simulink library "Px4Library"  (R2015b)
settings: Solver=VariableStepAuto  StartTime=0.0  StopTime=10.0  RelTol=1e-3
undefined symbols (not defined in the file): armed, ctrl_state, INIT_PARAM_VECTOR, mpc_att_sp, mpc_ctrl_state, mpc_manual, mpc_pos_sp_triplet, mpc_vehicle_land_detected, mpc_vehicle_status, v_att_sp, v_control_mode
libraries: simulink x4
(part 1 of 7)
settings Model: Creator=jeremiebannwarth  LastModifiedBy=jban039

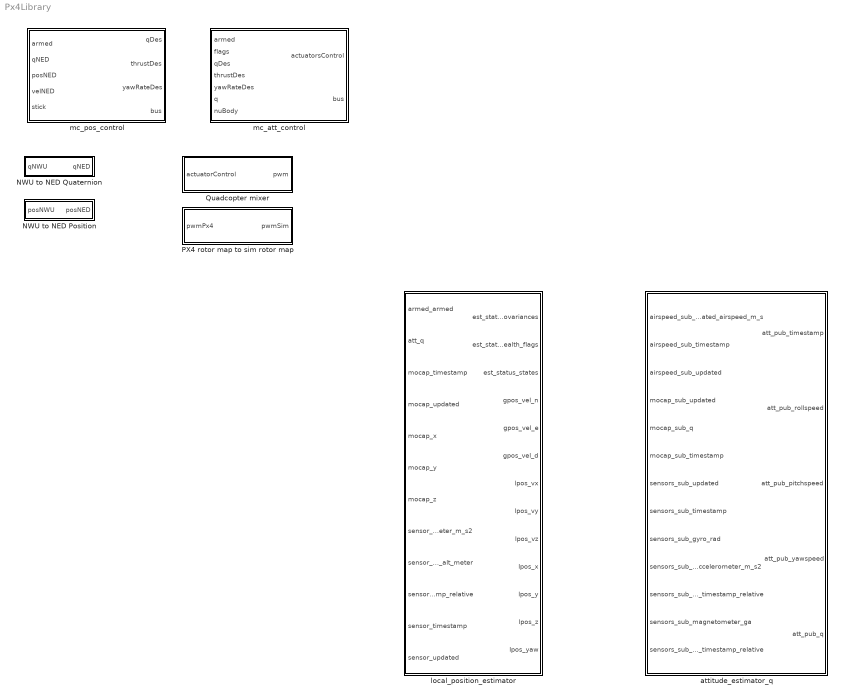
== system Px4Library ==
  NWU to NED Position : Subsystem  mask(Coordinate transform){}
      mask help:
      | Convert a 3x1 vector or 4x1 quaternion from a North West Up to a North East Down coordinate system.
      |
      | The appropriate coordinate transform is automatically selected based on the input size.
  NWU to NED Quaternion : Subsystem  mask(Coordinate transform){}
      mask help:
      | Convert a 3x1 vector or 4x1 quaternion from a North West Up to a North East Down coordinate system.
      |
      | The appropriate coordinate transform is automatically selected based on the input size.
  PX4 rotor map to sim rotor map : Subsystem
      mask Display:
      | disp(sprintf('MOTOR\nMAP'))
      | port_label('output', 1, sprintf('sim\npwm'))
      | port_label('input', 1, sprintf('px4\npwm'))
  Quadcopter mixer : Subsystem  mask{MC_SAMPLING_PERIOD=0.002}
      mask Display:
      | disp('MIXER')
      | port_label('input', 1, sprintf('actuators\ncontrol'))
      | port_label('output', 1, sprintf('px4\npwm'))
  attitude_estimator_q : Subsystem  mask(PX4 LPE (local position estimator): local_position_estimator){Q_SAMPLING_PERIOD=0.002, ATT_W_ACC=0.2, ATT_W_MAG=0.1, ATT_W_EXT_HDG=0.1, ATT_W_GYRO_BIAS=0.1, ATT_MAG_DECL=0, ATT_MAG_DECL_A=1, ATT_EXT_HDG_M=0, ATT_ACC_COMP=1, ATT_BIAS_MAX=0.05, FW_ARSP_MODE=0}
      mask prompts: Q_SAMPLING_PERIOD "Sampling period (s)"; ATT_W_ACC "ATT_W_ACC - Complimentary filter accelerometer weight (-)"; ATT_W_MAG "ATT_W_MAG - Complimentary filter magnetometer weight (-)"; ATT_W_EXT_HDG "ATT_W_EXT_HDG - Complimentary filter external heading weight (-)"; ATT_W_GYRO_BIAS "ATT_W_GYRO_BIAS - Complimentary filter gyroscope bias weight (-)"; ATT_MAG_DECL "ATT_MAG_DECL - Magnetic declination. Not used when GPS available (deg)"; ATT_MAG_DECL_A "ATT_MAG_DECL_A - Automatic GPS based declination compensation (-)"; ATT_EXT_HDG_M "ATT_EXT_HDG_M - External heading usage mode (from Motion capture/Vision) (-), 0 None 1 Vision 2 Motion Capture"; ATT_ACC_COMP "ATT_ACC_COMP - Acceleration compensation based on GPS velocity. (-)"; ATT_BIAS_MAX "ATT_BIAS_MAX - Gyro bias limit (rad/s)"; FW_ARSP_MODE "FW_ARSP_MODE - Method used to publish the airspeed (-), 0 Measured airspeed 1 Vehicle ground speed 2 Airspeed invalid"
      mask TypeOptions ATT_EXT_HDG_M: 0 | 1 | 2
      mask TypeOptions FW_ARSP_MODE: 0 | 1 | 2
  local_position_estimator : Subsystem  mask(PX4 LPE (local position estimator): local_position_estimator){LPE_SAMPLING_PERIOD=0.02, ATT_W_ACC=0.2, Barometer=off, GPS=off, LIDAR=off, Flow=off, Sonar=off, Vision=off, Mocap=off, Land=off}
      mask prompts: LPE_SAMPLING_PERIOD "Sampling period (s)"; ATT_W_ACC "ATT_W_ACC - Complimentary filter accelerometer weight (-)"; Barometer "Use Barometer"; GPS "Use GPS"; LIDAR "Use LIDAR"; Flow "Use Flow"; Sonar "Use Sonar"; Vision "Use Vision"; Mocap "Use Mocap"; Land "Use Land"
      mask Callback Barometer:
      | status = get_param( gcb, 'Barometer' );
      | if strcmp( status, 'on' )
      | 	lpe = bitor( uint8(str2num(get_param( gcb, 'LPE_FUSION' ))), uint8(2^0) );
      | 	set_param( gcb, 'LPE_FUSION', num2str(lpe) );
      | else
      | 	lpe = bitand( uint8(str2num(get_param( gcb, 'LPE_FUSION' ))), bitcmp(uint8(2^0), 'uint8' ));
      | 	set_param( gcb, 'LPE_FUSION', num2str(lpe) );
      | end
      mask Callback GPS:
      | status = get_param( gcb, 'GPS' );
      | if strcmp( status, 'on' )
      | 	lpe = bitor( uint8(str2num(get_param( gcb, 'LPE_FUSION' ))), uint8(2^1) );
      | 	set_param( gcb, 'LPE_FUSION', num2str(lpe) );
      | else
      | 	lpe = bitand( uint8(str2num(get_param( gcb, 'LPE_FUSION' ))), bitcmp(uint8(2^1), 'uint8' ));
      | 	set_param( gcb, 'LPE_FUSION', num2str(lpe) );
      | end
      mask Callback LIDAR:
      | status = get_param( gcb, 'LIDAR' );
      | if strcmp( status, 'on' )
      | 	lpe = bitor( uint8(str2num(get_param( gcb, 'LPE_FUSION' ))), uint8(2^2) );
      | 	set_param( gcb, 'LPE_FUSION', num2str(lpe) );
      | else
      | 	lpe = bitand( uint8(str2num(get_param( gcb, 'LPE_FUSION' ))), bitcmp(uint8(2^2), 'uint8' ));
      | 	set_param( gcb, 'LPE_FUSION', num2str(lpe) );
      | end
      mask Callback Flow:
      | status = get_param( gcb, 'Flow' );
      | if strcmp( status, 'on' )
      | 	lpe = bitor( uint8(str2num(get_param( gcb, 'LPE_FUSION' ))), uint8(2^3) );
      | 	set_param( gcb, 'LPE_FUSION', num2str(lpe) );
      | else
      | 	lpe = bitand( uint8(str2num(get_param( gcb, 'LPE_FUSION' ))), bitcmp(uint8(2^3), 'uint8' ));
      | 	set_param( gcb, 'LPE_FUSION', num2str(lpe) );
      | end
      mask Callback Sonar:
      | status = get_param( gcb, 'Sonar' );
      | if strcmp( status, 'on' )
      | 	lpe = bitor( uint8(str2num(get_param( gcb, 'LPE_FUSION' ))), uint8(2^4) );
      | 	set_param( gcb, 'LPE_FUSION', num2str(lpe) );
      | else
      | 	lpe = bitand( uint8(str2num(get_param( gcb, 'LPE_FUSION' ))), bitcmp(uint8(2^4), 'uint8' ));
      | 	set_param( gcb, 'LPE_FUSION', num2str(lpe) );
      | end
      mask Callback Vision:
      | status = get_param( gcb, 'Vision' );
      | if strcmp( status, 'on' )
      | 	lpe = bitor( uint8(str2num(get_param( gcb, 'LPE_FUSION' ))), uint8(2^5) );
      | 	set_param( gcb, 'LPE_FUSION', num2str(lpe) );
      | else
      | 	lpe = bitand( uint8(str2num(get_param( gcb, 'LPE_FUSION' ))), bitcmp(uint8(2^5), 'uint8' ));
      | 	set_param( gcb, 'LPE_FUSION', num2str(lpe) );
      | end
      mask Callback Mocap:
      | status = get_param( gcb, 'Mocap' );
      | if strcmp( status, 'on' )
      | 	lpe = bitor( uint8(str2num(get_param( gcb, 'LPE_FUSION' ))), uint8(2^6) );
      | 	set_param( gcb, 'LPE_FUSION', num2str(lpe) );
      | else
      | 	lpe = bitand( uint8(str2num(get_param( gcb, 'LPE_FUSION' ))), bitcmp(uint8(2^6), 'uint8' ));
      | 	set_param( gcb, 'LPE_FUSION', num2str(lpe) );
      | end
      mask Callback Land:
      | status = get_param( gcb, 'Land' );
      | if strcmp( status, 'on' )
      | 	lpe = bitor( uint8(str2num(get_param( gcb, 'LPE_FUSION' ))), uint8(2^7) );
      | 	set_param( gcb, 'LPE_FUSION', num2str(lpe) );
      | else
      | 	lpe = bitand( uint8(str2num(get_param( gcb, 'LPE_FUSION' ))), bitcmp(uint8(2^7), 'uint8' ));
      | 	set_param( gcb, 'LPE_FUSION', num2str(lpe) );
      | end
  mc_att_control : Subsystem  mask(PX4 Attitude Controller: mc_att_control){MC_SAMPLING_PERIOD=0.002, MC_ROLL_TC=0.2, MC_PITCH_TC=0.2, MC_ROLL_P=6.5, MC_ROLLRATE_P=0.15, MC_ROLLRATE_I=0.05, MC_ROLLRATE_D=0.003, MC_ROLLRATE_FF=0.0, MC_PITCH_P=6.5, MC_PITCHRATE_P=0.15, MC_PITCHRATE_I=0.05, MC_PITCHRATE_D=0.003, MC_PITCHRATE_FF=0.0, MC_YAW_P=2.8, MC_YAWRATE_P=0.2, MC_YAWRATE_I=0.1, MC_YAWRATE_D=0.0, MC_YAWRATE_FF=0.0, MC_YAW_FF=0.5, MC_ROLLRATE_MAX=220.0, MC_PITCHRATE_MAX=220.0, MC_YAWRATE_MAX=200.0, MC_YAWRAUTO_MAX=45.0, MC_ACRO_R_MAX=360.0, MC_ACRO_P_MAX=360.0, MC_ACRO_Y_MAX=360.0, MC_RATT_TH=0.8, MC_TPA_BREAK=1.0, MC_TPA_SLOPE=1.0, VT_OPT_RECOV_EN=0.0, VT_WV_YAWR_SCL=0.15, MC_RR_INT_LIM=0.30, MC_PR_INT_LIM=0.30, MC_TPA_BREAK_P=1.0, MC_TPA_BREAK_I=1.0, MC_TPA_BREAK_D=1.0, MC_TPA_RATE_P=0.0, MC_TPA_RATE_I=0.0, MC_TPA_RATE_D=0.0, VT_TYPE=2.0, MC_BAT_SCALE_EN=0.0, MC_YR_INT_LIM=0.30}
      mask prompts: VT_TYPE "VT_TYPE (0 = Tailsitter, 1 = Tiltrotor, 2 = Standard)"
      mask help: Stabilization controller from the PX4 flight stack.
  mc_pos_control : Subsystem  mask{THROTTLE_HOVER=0.61703684833922, MPC_SAMPLING_PERIOD=0.02, MPC_THR_MIN=0.12, MPC_THR_HOVER=0.5, MPC_ALTCTL_DZ=0.1, MPC_ALTCTL_DY=0.0, MPC_THR_MAX=0.9, MPC_MANTHR_MIN=0.08, MPC_MANTHR_MAX=0.9, MPC_Z_P=1.0, MPC_Z_VEL_P=0.2, MPC_Z_VEL_I=0.02, MPC_Z_VEL_D=0.0, MPC_Z_VEL_MAX_UP=3.0, MPC_Z_VEL_MAX=1.0, MPC_Z_VEL_MAX_DN=1.0, MPC_Z_FF=0.5, MPC_XY_P=0.95, MPC_XY_VEL_P=0.09, MPC_XY_VEL_I=0.02, MPC_XY_VEL_D=0.01, MPC_XY_CRUISE=5.0, MPC_XY_VEL_MAX=8.0, MPC_XY_FF=0.5, MPC_TILTMAX_AIR=45.0, MPC_TILTMAX_LND=12.0, MPC_LAND_SPEED=0.5, MPC_TKO_SPEED=1.5, MPC_MAN_R_MAX=35.0, MPC_MAN_P_MAX=35.0, MPC_MAN_Y_MAX=200.0, MPC_HOLD_XY_DZ=0.1, MPC_HOLD_MAX_XY=0.8, MPC_HOLD_MAX_Z=0.6, MPC_VELD_LP=5.0, MPC_ACC_HOR_MAX=5.0, MPC_ALT_MODE=0, MC_YAWRATE_MAX=200.0, MC_YAW_P=2.8, VT_OPT_RECOV_EN=0}
      mask init:
      | throttle_hover = THROTTLE_HOVER; % evalin('base', THROTTLE_HOVER);
      | MPC_INIT_SELF = struct( 'mpc_param_find', struct( ...
      | 'MC_YAWRATE_MAX', str2num(MC_YAWRATE_MAX), ...
      | 'MC_YAW_P', str2num(MC_YAW_P), ...
      | 'MPC_ACC_HOR_MAX', str2num(MPC_ACC_HOR_MAX), ...
      | 'MPC_ALTCTL_DY', str2num(MPC_ALTCTL_DY), ...
      | 'MPC_ALTCTL_DZ', str2num(MPC_ALTCTL_DZ), ...
      | 'MPC_ALT_MODE', str2num(MPC_ALT_MODE), ...
      | 'MPC_HOLD_MAX_XY', str2num(MPC_HOLD_MAX_XY), ...
      | 'MPC_HOLD_MAX_Z', str2num(MPC_HOLD_MAX_Z), ...
      | 'MPC_HOLD_XY_DZ', str2num(MPC_HOLD_XY_DZ), ...
      | 'MPC_LAND_SPEED', str2num(MPC_LAND_SPEED), ...
      | 'MPC_MAN_P_MAX', str2num(MPC_MAN_P_MAX), ...
      | 'MPC_MAN_R_MAX', str2num(MPC_MAN_R_MAX), ...
      | 'MPC_MAN_Y_MAX', str2num(MPC_MAN_Y_MAX), ...
      | 'MPC_THR_HOVER', str2num(MPC_THR_HOVER), ...
      | 'MPC_THR_MAX', str2num(MPC_THR_MAX), ...
      | 'MPC_THR_MIN', str2num(MPC_THR_MIN), ...
      | 'MPC_TILTMAX_AIR', str2num(MPC_TILTMAX_AIR), ...
      | 'MPC_TILTMAX_LND', str2num(MPC_TILTMAX_LND), ...
      | 'MPC_TKO_SPEED', str2num(MPC_TKO_SPEED), ...
      | 'MPC_XY_CRUISE', str2num(MPC_XY_CRUISE), ...
      | 'MPC_XY_FF', str2num(MPC_XY_FF), ...
      | 'MPC_XY_P', str2num(MPC_XY_P), ...
      | 'MPC_XY_VEL_D', str2num(MPC_XY_VEL_D), ...
      | 'MPC_XY_VEL_I', str2num(MPC_XY_VEL_I), ...
      | 'MPC_XY_VEL_MAX', str2num(MPC_XY_VEL_MAX), ...
      | 'MPC_XY_VEL_P', str2num(MPC_XY_VEL_P), ...
      | 'MPC_Z_FF', str2num(MPC_Z_FF), ...
      | 'MPC_Z_P', str2num(MPC_Z_P), ...
      | 'MPC_Z_VEL_D', str2num(MPC_Z_VEL_D), ...
      | 'MPC_Z_VEL_I', str2num(MPC_Z_VEL_I), ...
      | 'MPC_Z_VEL_MAX', str2num(MPC_Z_VEL_MAX), ...
      | 'MPC_Z_VEL_MAX_DN', str2num(MPC_Z_VEL_MAX_DN), ...
      | 'MPC_Z_VEL_MAX_UP', str2num(MPC_Z_VEL_MAX_UP), ...
      | 'MPC_Z_VEL_P', str2num(MPC_Z_VEL_P), ...
      | 'VT_OPT_RECOV_EN', str2num(VT_OPT_RECOV_EN), ...
      | 'MPC_VELD_LP', str2num(MPC_VELD_LP) ...
      | ), ...
      | 'mpc_thrust_int', [0; 0; -throttle_hover], ...
      | 'mpc_att_sp', struct('thrust', throttle_hover, ...
      | 'q_d', [1; 0; 0; 0;]) ...
      | );

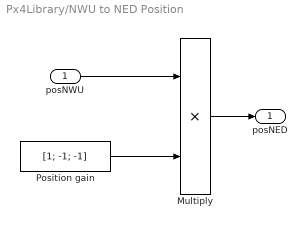
== system Px4Library/NWU to NED Position ==
  posNWU : Inport
  Multiply : Product  Inputs=**
  Position gain : Constant  Value=[1; -1; -1]
  posNED : Outport
  wires:
  Position gain/1 -> Multiply/2
  Multiply/1 -> posNED/1
  posNWU/1 -> Multiply/1

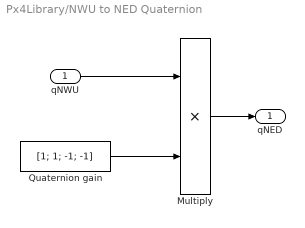
== system Px4Library/NWU to NED Quaternion ==
  qNWU : Inport
  Multiply : Product  Inputs=**
  Quaternion gain : Constant  Value=[1; 1; -1; -1]
  qNED : Outport
  wires:
  qNWU/1 -> Multiply/1
  Multiply/1 -> qNED/1
  Quaternion gain/1 -> Multiply/2

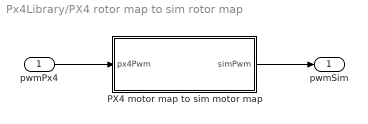
== system Px4Library/PX4 rotor map to sim rotor map ==
  pwmPx4 : Inport
  PX4 motor map to sim motor map : MATLAB Function  TreatAsAtomicUnit=on
  pwmSim : Outport
  wires:
  PX4 motor map to sim motor map/1(simPwm) -> pwmSim/1
  pwmPx4/1 -> PX4 motor map to sim motor map/1(px4Pwm)

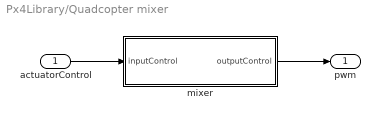
== system Px4Library/Quadcopter mixer ==
  actuatorControl : Inport
  mixer : MATLAB Function  TreatAsAtomicUnit=on  SystemSampleTime=MC_SAMPLING_PERIOD
  pwm : Outport
  wires:
  actuatorControl/1 -> mixer/1(inputControl)
  mixer/1(outputControl) -> pwm/1

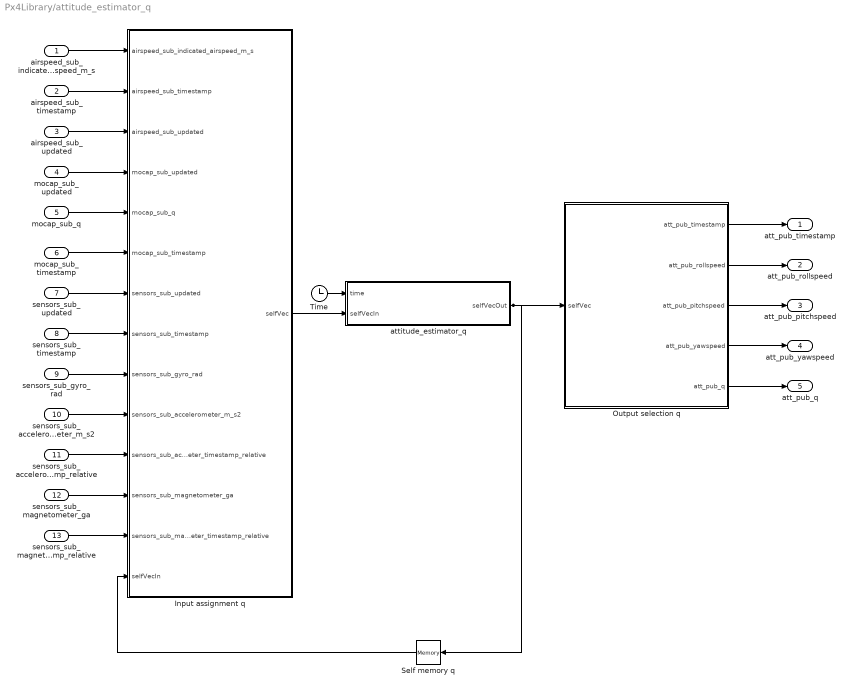
== system Px4Library/attitude_estimator_q ==
  airspeed_sub_indicated_airspeed_m_s : Inport
  airspeed_sub_timestamp : Inport  Port=2
  airspeed_sub_updated : Inport  Port=3
  mocap_sub_updated : Inport  Port=4
  mocap_sub_q : Inport  Port=5
  mocap_sub_timestamp : Inport  Port=6
  sensors_sub_updated : Inport  Port=7
  sensors_sub_timestamp : Inport  Port=8
  sensors_sub_gyro_rad : Inport  Port=9
  sensors_sub_accelerometer_m_s2 : Inport  Port=10
  sensors_sub_accelerometer_timestamp_relative : Inport  Port=11
  sensors_sub_magnetometer_ga : Inport  Port=12
  sensors_sub_magnetometer_timestamp_relative : Inport  Port=13
  Input assignment q : MATLAB Function  TreatAsAtomicUnit=on
  Output selection q : MATLAB Function  TreatAsAtomicUnit=on
  Self memory q : Memory  X0=[ATT_ACC_COMP, 0, 0, 0, 0, 0, 0, FW_ARSP_MODE, 0, 0, 0, 0, 0, 0, 0, 0, 0, 0, 0, ATT_BIAS_MAX, 0, 0, 0, 0, 0, 0, 0, 0, 0, 0, 0, 0, 0, 0, 0, 0, 0, 0, 0.02, 0, ATT_EXT_HDG_M, 0, 0, 0, 0, 0, 0, 0, 0, 0, 0, 0, 0, 0, 0, 0, 0, 0, 0, 0, 0, 0, 0, 0, 0, 0, 0, 0, 0, 0, 0, 0, 0, 0, 0, 0, 0, 0, 0, 0, 0, 0, 0, 0, 0, 0, 0, 0, 0, 0, 0, 0, 0, 0, 0, 0, 0, 0, 0, 0, 0, 0, 0, 0, 0, 0, 0, 0, 0, 0, 0, 0, 0, 0, 0, 0, 0, 0, 0, 0, 0, 0, ATT_MAG_DECL, ATT_MAG_DECL_A, 0, 0, 0, 0, 0, 0, 0, 0, 0, 0, 0, 0, 0, 0, 0, 0, 0, 0, 0, 0, 0, 0, 0, 0, 0, 0, 0, 0, 0, 0, 0, 0, 0, 0, 0, 0, 0, 0, 0, 0, 0, 0, 0, 0, 0, 0, 0, 0, 0, 0, 0, 0, 0, 0, 0, 0, 0, 0, 0, 0, ATT_W_ACC, ATT_W_EXT_HDG, ATT_W_GYRO_BIAS, ATT_W_MAG, 0, 0]
  Time : Clock
  attitude_estimator_q : MATLAB Function  TreatAsAtomicUnit=on  SystemSampleTime=Q_SAMPLING_PERIOD
  att_pub_timestamp : Outport
  att_pub_rollspeed : Outport  Port=2
  att_pub_pitchspeed : Outport  Port=3
  att_pub_yawspeed : Outport  Port=4
  att_pub_q : Outport  Port=5
  wires:
  Input assignment q/1(selfVec) -> attitude_estimator_q/2(selfVecIn)
  attitude_estimator_q/1(selfVecOut) -> Output selection q/1(selfVec), Self memory q/1
  Self memory q/1 -> Input assignment q/14(selfVecIn)
  Time/1 -> attitude_estimator_q/1(time)
  airspeed_sub_indicated_airspeed_m_s/1 -> Input assignment q/1(airspeed_sub_indicated_airspeed_m_s)
  airspeed_sub_timestamp/1 -> Input assignment q/2(airspeed_sub_timestamp)
  airspeed_sub_updated/1 -> Input assignment q/3(airspeed_sub_updated)
  mocap_sub_updated/1 -> Input assignment q/4(mocap_sub_updated)
  mocap_sub_q/1 -> Input assignment q/5(mocap_sub_q)
  mocap_sub_timestamp/1 -> Input assignment q/6(mocap_sub_timestamp)
  sensors_sub_updated/1 -> Input assignment q/7(sensors_sub_updated)
  sensors_sub_timestamp/1 -> Input assignment q/8(sensors_sub_timestamp)
  sensors_sub_gyro_rad/1 -> Input assignment q/9(sensors_sub_gyro_rad)
  sensors_sub_accelerometer_m_s2/1 -> Input assignment q/10(sensors_sub_accelerometer_m_s2)
  sensors_sub_accelerometer_timestamp_relative/1 -> Input assignment q/11(sensors_sub_accelerometer_timestamp_relative)
  sensors_sub_magnetometer_ga/1 -> Input assignment q/12(sensors_sub_magnetometer_ga)
  sensors_sub_magnetometer_timestamp_relative/1 -> Input assignment q/13(sensors_sub_magnetometer_timestamp_relative)
  Output selection q/1(att_pub_timestamp) -> att_pub_timestamp/1
  Output selection q/2(att_pub_rollspeed) -> att_pub_rollspeed/1
  Output selection q/3(att_pub_pitchspeed) -> att_pub_pitchspeed/1
  Output selection q/4(att_pub_yawspeed) -> att_pub_yawspeed/1
  Output selection q/5(att_pub_q) -> att_pub_q/1

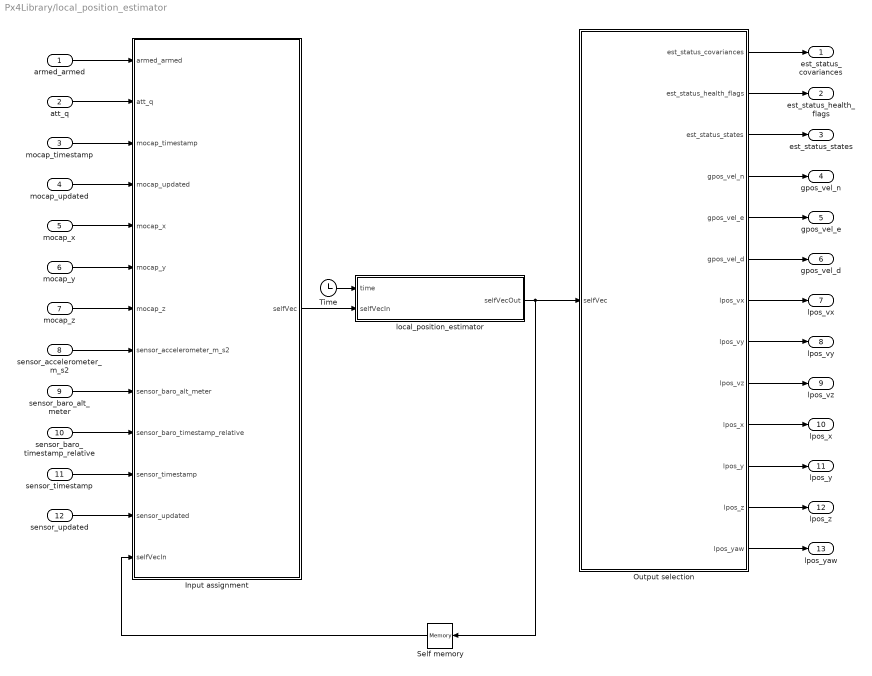
== system Px4Library/local_position_estimator ==
  armed_armed : Inport
  att_q : Inport  Port=2
  mocap_timestamp : Inport  Port=3
  mocap_updated : Inport  Port=4
  mocap_x : Inport  Port=5
  mocap_y : Inport  Port=6
  mocap_z : Inport  Port=7
  sensor_accelerometer_m_s2 : Inport  Port=8
  sensor_baro_alt_meter : Inport  Port=9
  sensor_baro_timestamp_relative : Inport  Port=10
  sensor_timestamp : Inport  Port=11
  sensor_updated : Inport  Port=12
  Input assignment : MATLAB Function  TreatAsAtomicUnit=on
  Output selection : MATLAB Function  TreatAsAtomicUnit=on
  Self memory : Memory  X0=[0, 0, 0, 0, 0, 0, 0, 0, 0, 0, 0, 0, 0, 0, 0, 0, 0, 0, 0, 0, 0, 0, 0, 0, 0, 0, 0, 0, 0, 0, 0, 0, 0, 0, 0, 0, 0, 0, 0, 0, 0, 0, 0, 0, 0, 0, 0, 0, 0, 0, 0, 0, 0, 0, 0, 0, 0, 0, 0, 0, 0, 0, 0, 0, 0, 0, 0, 0, 0, 0, 0, 0, 0, 0, 0, 0, 0, 0, 0, 0, 0, 0, 0, 0, 0, 0, 0, 0, 0, 0, 0, 0, 0, 0, 0, 0, 0, 0, 0, 0, 0, 0, 0, 0, 0, 0, 0, 0, 0, 0, 0, 0, 0, 0, 0, 0, 0, 0, 0, 0, 0, 0, 0, 0, 0, 0, 0, 0, 0, 0, 0, 8.82050518214, 12.094592431, 13.9876612368, 16.0875642296, 17.8797700658, 19.6465647819, 1e-1, 2.0, 2.0, 2.0, 2^2, 2^0, 2^1, 2^7, 2^1, 2^6, 2^0, 2^4, 2^5, 2^2, 2^3, 0, 10.0, 8, 0, 0, 0, 0, 0, 0, 0, 0, 0, 0, 8, 0, 0, 0, 0, 0, 0, 0, 0, 0, 0, 8, 0, 0, 0, 0, 0, 0, 0, 0, 0, 0, 2*LPE_VXY_PUB*LPE_VXY_PUB, 0, 0, 0, 0, 0, 0, 0, 0, 0, 0, 2*LPE_VXY_PUB*LPE_VXY_PUB, 0, 0, 0, 0, 0, 0, 0, 0, 0, 0, 2*LPE_VXY_PUB*LPE_VXY_PUB, 0, 0, 0, 0, 0, 0, 0, 0, 0, 0, 1e-6, 0, 0, 0, 0, 0, 0, 0, 0, 0, 0, 1e-6, 0, 0, 0, 0, 0, 0, 0, 0, 0, 0, 1e-6, 0, 0, 0, 0, 0, 0, 0, 0, 0, 0, 8, 1.0e6, 0, 0, 0, 0, 0, 0, 0, 0, 0, 0, 0, 0, 0, 0, 0, 0, 0, 0, 0, 0, 0, 0, 0, 0, 0, 0, 0, 0, 0, 0, 0, 0, 0, 0, 0, 0, 0, 0, 0, 0, 0, 0, 0, 0, 0, 0, 0, 0, 0, 0, 0, 0, 0, 0, 0, 0, 0, 0, 0, 0, 0, 0, 0, 0, 0, 0, 0, 0, 0, 0, 0, 0, 0, 0, 0, 0, 0, 0, 0, 0, 0, 0, 0, 0, 0, 0, 0, 0, 0, 0, 0, 0, 0, 0, 0, 0, 0, 0, 0, 0, 0, 0, 0, 0, 0, 0, 0, 0, 0, 0, 0, 0, 0, 0, 0, 0, 0, 0, 2^0, 2^3, 2^1, 2^7, 2^2, 2^6, 2^4, 2^5, 0, LPE_ACC_XY, 0, LPE_ACC_Z, LPE_SAMPLING_PERIOD, LPE_X_LP, 0, 0, 0, 0, 0, 0, LPE_BAR_Z, LPE_SAMPLING_PERIOD, 0, 0, 0, 0, LPE_FAKE_ORIGIN, 0, LPE_FGYRO_HP, LPE_FGYRO_HP, LPE_FLW_QMIN, LPE_FLW_R, LPE_FLW_RR, LPE_FLW_SCALE, LPE_FLW_OFF_Z, LPE_FUSION, 0, LPE_GPS_DELAY, LPE_EPH_MAX, LPE_EPV_MAX, LPE_GPS_VXY, LPE_GPS_VZ, LPE_GPS_XY, LPE_GPS_Z, LPE_LAT, LPE_LON, 0, 0, LPE_LAND_VXY, LPE_LAND_Z, 0, LPE_LDR_OFF_Z, LPE_LDR_Z, 0, 0, 0, 0, 0, 0, 0, LPE_VIC_P, LPE_PN_B, LPE_PN_P, LPE_PN_T, LPE_PN_V, 8, 0, 0, 0, 0, 0, 0, 0, 0, 0, 0, 0, 0, 0, 0, 0, 0, 0, 0, 0, 0, 0, 0, 0, 0, 0, 0, 0, 0, 0, 0, 0, 0, 0, 0, 0, 0, 0, 0, 0, 0, 0, 0, 0, 0, 0, 0, 0, 0, 0, 0, 0, 0, 0, 0, 0, 0, 0, 0, 0, 0, 0, 0, 0, 0, 0, 0, 0, 0, 0, 0, 0, 0, 0, 0, 255, 0, LPE_SNR_OFF_Z, LPE_SNR_Z, 0, 0, 0, 0, 0, 0, 0, 0, 0, 0, 0, 0, 0, 0, 0, 0, 0, 0, 0, 0, 0, 0, 0, 0, 0, 0, 0, 0, 0, 0, 0, 0, 0, 0, 0, 0, 0, 0, 0, 1, 1, LPE_T_MAX_GRADE, 0, 0, 0, 0, 0, 0, 0, 0, 0, 0, 0, LPE_VIS_DELAY, LPE_VIS_XY, LPE_VIS_Z, LPE_VXY_PUB, 0, 0, 0, 0, 0, 0, 0, 0, 0, 0, 0, 0, 0, 0, 0, 0, 0, 0, 0, 0, 0, 0, 0, 0, 0, 0, 0, 0, 0, 0, 0, 0, 0, 0, 0, 0, 0, 0, 0, 0, 0, 0, 0, 0, 0, 0, 0, 0, 0, 0, 0, 0, 0, 0, 0, 0, 0, 0, 0, 0, 0, 0, 0, 0, 0, 0, 0, 0, 0, 0, 0, 0, 0, 0, 0, 0, 0, 0, 0, 0, 0, 0, 0, 0, 0, 0, 0, 0, 0, 0, 0, 0, 0, 0, 0, 0, 0, 0, 0, 0, 0, 0, 0, 0, 0, 0, 0, 0, 0, 0, 1, 1, LPE_SAMPLING_PERIOD, LPE_X_LP, 0, 0, 0, 0, 0, 0, 0, 0, 0, 0, LPE_Z_PUB]
  Time : Clock
  local_position_estimator : MATLAB Function  TreatAsAtomicUnit=on  SystemSampleTime=LPE_SAMPLING_PERIOD
  est_status_covariances : Outport
  est_status_health_flags : Outport  Port=2
  est_status_states : Outport  Port=3
  gpos_vel_n : Outport  Port=4
  gpos_vel_e : Outport  Port=5
  gpos_vel_d : Outport  Port=6
  lpos_vx : Outport  Port=7
  lpos_vy : Outport  Port=8
  lpos_vz : Outport  Port=9
  lpos_x : Outport  Port=10
  lpos_y : Outport  Port=11
  lpos_z : Outport  Port=12
  lpos_yaw : Outport  Port=13
  wires:
  Input assignment/1(selfVec) -> local_position_estimator/2(selfVecIn)
  local_position_estimator/1(selfVecOut) -> Output selection/1(selfVec), Self memory/1
  Self memory/1 -> Input assignment/13(selfVecIn)
  Time/1 -> local_position_estimator/1(time)
  armed_armed/1 -> Input assignment/1(armed_armed)
  att_q/1 -> Input assignment/2(att_q)
  mocap_timestamp/1 -> Input assignment/3(mocap_timestamp)
  mocap_updated/1 -> Input assignment/4(mocap_updated)
  mocap_x/1 -> Input assignment/5(mocap_x)
  mocap_y/1 -> Input assignment/6(mocap_y)
  mocap_z/1 -> Input assignment/7(mocap_z)
  sensor_accelerometer_m_s2/1 -> Input assignment/8(sensor_accelerometer_m_s2)
  sensor_baro_alt_meter/1 -> Input assignment/9(sensor_baro_alt_meter)
  sensor_baro_timestamp_relative/1 -> Input assignment/10(sensor_baro_timestamp_relative)
  sensor_timestamp/1 -> Input assignment/11(sensor_timestamp)
  sensor_updated/1 -> Input assignment/12(sensor_updated)
  Output selection/1(est_status_covariances) -> est_status_covariances/1
  Output selection/2(est_status_health_flags) -> est_status_health_flags/1
  Output selection/3(est_status_states) -> est_status_states/1
  Output selection/4(gpos_vel_n) -> gpos_vel_n/1
  Output selection/5(gpos_vel_e) -> gpos_vel_e/1
  Output selection/6(gpos_vel_d) -> gpos_vel_d/1
  Output selection/7(lpos_vx) -> lpos_vx/1
  Output selection/8(lpos_vy) -> lpos_vy/1
  Output selection/9(lpos_vz) -> lpos_vz/1
  Output selection/10(lpos_x) -> lpos_x/1
  Output selection/11(lpos_y) -> lpos_y/1
  Output selection/12(lpos_z) -> lpos_z/1
  Output selection/13(lpos_yaw) -> lpos_yaw/1

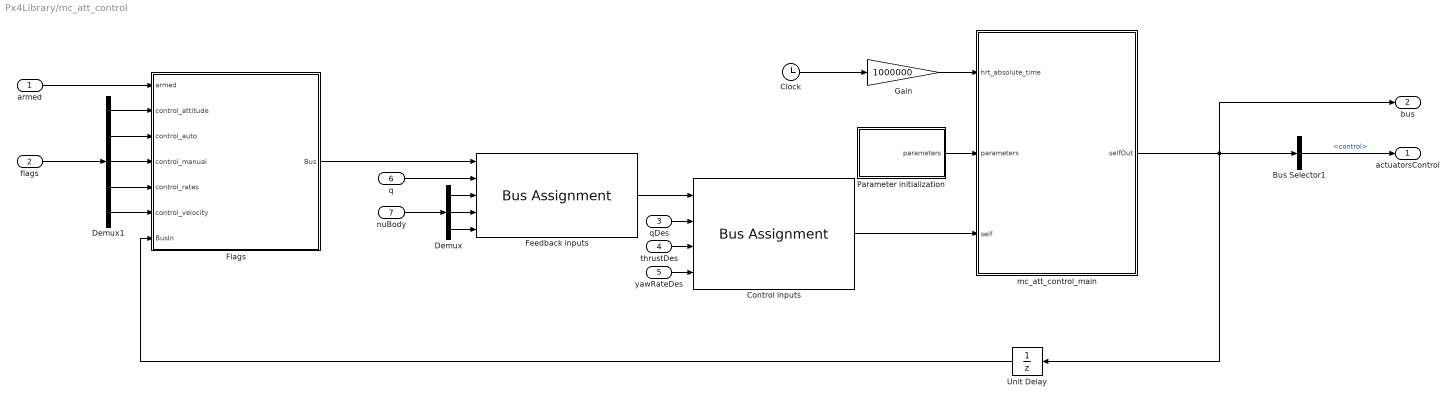
== system Px4Library/mc_att_control ==
  armed : Inport  PortDimensions=1  SampleTime=MC_SAMPLING_PERIOD
  flags : Inport  Port=2  PortDimensions=5  SampleTime=MC_SAMPLING_PERIOD
  qDes : Inport  Port=3  PortDimensions=4  SampleTime=MC_SAMPLING_PERIOD
  thrustDes : Inport  Port=4  PortDimensions=1  SampleTime=MC_SAMPLING_PERIOD
  yawRateDes : Inport  Port=5  PortDimensions=1  SampleTime=MC_SAMPLING_PERIOD
  q : Inport  Port=6  PortDimensions=4  SampleTime=MC_SAMPLING_PERIOD
  nuBody : Inport  Port=7  PortDimensions=3  SampleTime=MC_SAMPLING_PERIOD
  Bus Selector1 : BusSelector  OutputSignals=actuators.control
  Clock : Clock
  Control inputs : BusAssignment  AssignedSignals=v_att_sp.q_d,v_att_sp.thrust,v_att_sp.yaw_sp_move_rate
  Demux : Demux  Outputs=3
  Demux1 : Demux  Outputs=5
  Feedback inputs : BusAssignment  AssignedSignals=ctrl_state.q,ctrl_state.roll_rate,ctrl_state.pitch_rate,ctrl_state.yaw_rate
  Flags : Subsystem
  Gain : Gain  Gain=1000000
  Parameter initialization : Subsystem
  Unit Delay : UnitDelay  SampleTime=MC_SAMPLING_PERIOD
  mc_att_control_main : MATLAB Function  TreatAsAtomicUnit=on  SystemSampleTime=MC_SAMPLING_PERIOD
  actuatorsControl : Outport  SampleTime=MC_SAMPLING_PERIOD
  bus : Outport  Port=2  SampleTime=MC_SAMPLING_PERIOD
  wires:
  mc_att_control_main/1(selfOut) -> bus/1, Unit Delay/1, Bus Selector1/1
  Parameter initialization/1(parameters) -> mc_att_control_main/2(parameters)
  Bus Selector1/1 -> actuatorsControl/1  "<control>"
  Unit Delay/1 -> Flags/7(BusIn)
  Control inputs/1 -> mc_att_control_main/3(self)
  Flags/1(Bus) -> Feedback inputs/1
  Demux/1 -> Feedback inputs/3
  Demux/2 -> Feedback inputs/4
  Demux/3 -> Feedback inputs/5
  Clock/1 -> Gain/1
  Gain/1 -> mc_att_control_main/1(hrt_absolute_time)
  Feedback inputs/1 -> Control inputs/1
  qDes/1 -> Control inputs/2
  thrustDes/1 -> Control inputs/3
  yawRateDes/1 -> Control inputs/4
  Demux1/5 -> Flags/6(control_velocity)
  Demux1/4 -> Flags/5(control_rates)
  Demux1/3 -> Flags/4(control_manual)
  Demux1/2 -> Flags/3(control_auto)
  Demux1/1 -> Flags/2(control_attitude)
  armed/1 -> Flags/1(armed)
  q/1 -> Feedback inputs/2
  nuBody/1 -> Demux/1
  flags/1 -> Demux1/1

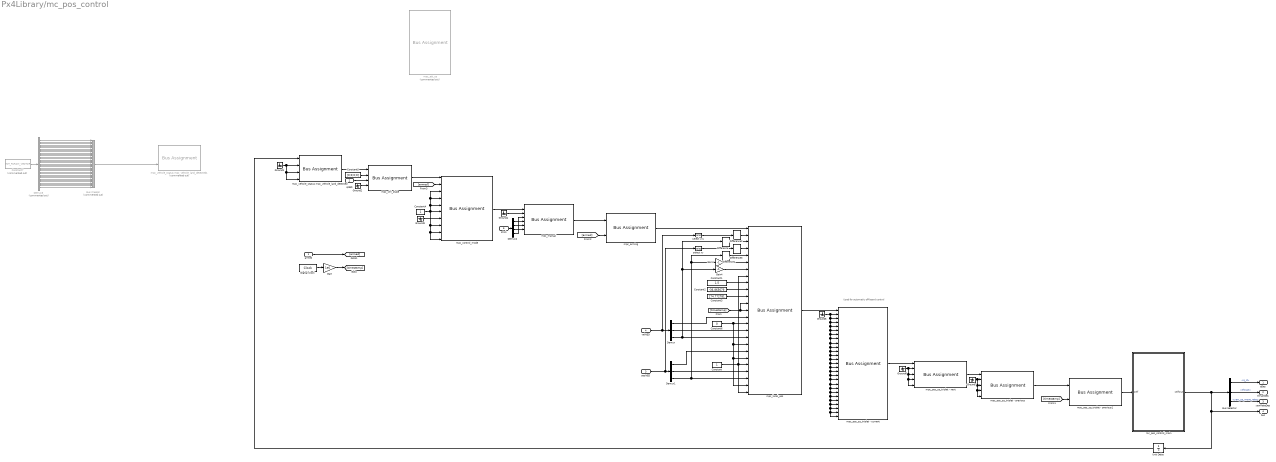
== system Px4Library/mc_pos_control ==
  note: Used for automatic off-board control
  armed : Inport  PortDimensions=1  SampleTime=MPC_SAMPLING_PERIOD
  qNED : Inport  Port=2  PortDimensions=4  SampleTime=MPC_SAMPLING_PERIOD
  posNED : Inport  Port=3  PortDimensions=3  SampleTime=MPC_SAMPLING_PERIOD
  velNED : Inport  Port=4  PortDimensions=3  SampleTime=MPC_SAMPLING_PERIOD
  stick : Inport  Port=5  PortDimensions=4  SampleTime=MPC_SAMPLING_PERIOD
  Bus Creator : BusCreator  Commented=on  Inputs=35  OutDataTypeStr=Bus: mpc_param_find
  Bus Selector : BusSelector  OutputSignals=mpc_att_sp.q_d,mpc_att_sp.thrust,mpc_att_sp.yaw_sp_move_rate
  Constant : Constant  SampleTime=MPC_SAMPLING_PERIOD
  Constant1 : Constant  Value=1.5  SampleTime=MPC_SAMPLING_PERIOD
  Constant2 : Constant  Value=-36.865679  SampleTime=MPC_SAMPLING_PERIOD
  Constant3 : Constant  Value=174.772781  SampleTime=MPC_SAMPLING_PERIOD
  Constant4 : Constant
  Constant5 : Constant  Value=[0;0;0;0]
  Constant6 : Constant  Value=0  SampleTime=MPC_SAMPLING_PERIOD
  Constant7 : Constant  Commented=on  Value=INIT_PARAM_VECTOR
  Demux : Demux  Outputs=3
  Demux1 : Demux  Outputs=3
  Demux2 : Demux
  Demux3 : Demux  Commented=on  Outputs=35
  Difference{,1..3} (4 alike) : simulink/Discrete/Difference  ICPrevInput=0.0  InputProcessing=Inherited  OutMin=[]  OutMax=[]  OutDataType=fixdt(1, 16)  OutScaling=2^-10  DoSatur=off
  Digital Clock : DigitalClock  SampleTime=MPC_SAMPLING_PERIOD
  Gain : Gain  Gain=1e6
  Gain1 : Gain  Gain=-1
  Gain4 : Gain  Gain=-1
  Ground{1..7} (7 alike) : Ground
  Unit Delay : UnitDelay  InitialCondition=MPC_INIT_SELF  SampleTime=MPC_SAMPLING_PERIOD
  mc_pos_control_main : MATLAB Function  TreatAsAtomicUnit=on  SystemSampleTime=MPC_SAMPLING_PERIOD
  mpc_arming : BusAssignment  AssignedSignals=mpc_arming.armed
  mpc_att_sp : BusAssignment  Commented=on  AssignedSignals=mpc_att_sp.disable_mc_yaw_control,mpc_att_sp.landing_gear,mpc_att_sp.pitch_body,mpc_att_sp.q_d,mpc_att_sp.q_d_valid,mpc_att_sp.roll_body,mpc_att_sp.thrust,mpc_att_sp.timestamp,mpc_att_sp.yaw_body,mpc_att_sp.yaw_sp_move_rate
  mpc_control_mode : BusAssignment  AssignedSignals=mpc_control_mode.flag_armed,mpc_control_mode.flag_control_acceleration_enabled,mpc_control_mode.flag_control_altitude_enabled,mpc_control_mode.flag_control_climb_rate_enabled,mpc_control_mode.flag_control_manual_enabled,mpc_control_mode.flag_control_offboard_enabled,mpc_control_mode.flag_control_position_enabled,mpc_control_mode.flag_control_velocity_enabled,mpc_control_mode.flag_control_attitude_enabled
  mpc_ctrl_state : BusAssignment  AssignedSignals=mpc_ctrl_state.delta_q_reset,mpc_ctrl_state.q,mpc_ctrl_state.quat_reset_counter
  mpc_local_pos : BusAssignment  AssignedSignals=mpc_local_pos.delta_vxy,mpc_local_pos.delta_vz,mpc_local_pos.delta_xy,mpc_local_pos.delta_z,mpc_local_pos.dist_bottom,mpc_local_pos.dist_bottom_rate,mpc_local_pos.dist_bottom_valid,mpc_local_pos.ref_alt,mpc_local_pos.ref_lat,mpc_local_pos.ref_lon,mpc_local_pos.ref_timestamp,mpc_local_pos.timestamp,mpc_local_pos.vx,mpc_local_pos.vxy_reset_counter,mpc_local_pos.vy,mpc_local_pos.vz,mpc_local_pos.vz_reset_counter,mpc_local_pos.x,mpc_local_pos.xy_reset_counter,mpc_local_pos.xy_valid,mpc_local_pos.y,mpc_local_pos.z,mpc_local_pos.z_reset_counter,mpc_local_pos.z_valid
  mpc_manual : BusAssignment  AssignedSignals=mpc_manual.gear_switch,mpc_manual.r,mpc_manual.x,mpc_manual.y,mpc_manual.z
  mpc_pos_sp_triplet - current : BusAssignment  AssignedSignals=mpc_pos_sp_triplet.mpc_current.a_x,mpc_pos_sp_triplet.mpc_current.a_y,mpc_pos_sp_triplet.mpc_current.a_z,mpc_pos_sp_triplet.mpc_current.acceleration_valid,mpc_pos_sp_triplet.mpc_current.acceptance_radius,mpc_pos_sp_triplet.mpc_current.alt,mpc_pos_sp_triplet.mpc_current.alt_valid,mpc_pos_sp_triplet.mpc_current.cruising_speed,mpc_pos_sp_triplet.mpc_current.disable_mc_yaw_control,mpc_pos_sp_triplet.mpc_current.lat,mpc_pos_sp_triplet.mpc_current.lon,mpc_pos_sp_triplet.mpc_current.position_valid,mpc_pos_sp_triplet.mpc_current.type,mpc_pos_sp_triplet.mpc_current.valid,mpc_pos_sp_triplet.mpc_current.velocity_frame,mpc_pos_sp_triplet.mpc_current.velocity_valid,mpc_pos_sp_triplet.mpc_current.vx,mpc_pos_sp_triplet.mpc_current.vy,mpc_pos_sp_triplet.mpc_current.vz,mpc_pos_sp_triplet.mpc_current.x,mpc_pos_sp_triplet.mpc_current.y,mpc_pos_sp_triplet.mpc_current.yaw,mpc_pos_sp_triplet.mpc_current.yaw_valid,mpc_pos_sp_triplet.mpc_current.yawspeed,mpc_pos_sp_triplet.mpc_current.yawspeed_valid,mpc_pos_sp_triplet.mpc_current.z
  mpc_pos_sp_triplet - next : BusAssignment  AssignedSignals=mpc_pos_sp_triplet.mpc_next.alt,mpc_pos_sp_triplet.mpc_next.lat,mpc_pos_sp_triplet.mpc_next.lon,mpc_pos_sp_triplet.mpc_next.valid
  mpc_pos_sp_triplet - previous : BusAssignment  AssignedSignals=mpc_pos_sp_triplet.mpc_previous.alt,mpc_pos_sp_triplet.mpc_previous.lat,mpc_pos_sp_triplet.mpc_previous.lon,mpc_pos_sp_triplet.mpc_previous.valid
  mpc_pos_sp_triplet - previous1 : BusAssignment  AssignedSignals=mpc_hrt_absolute_time
  mpc_vehicle_status mpc_vehicle_land_detected : BusAssignment  AssignedSignals=mpc_vehicle_status.is_rotary_wing,mpc_vehicle_status.is_vtol,mpc_vehicle_land_detected.landed
  mpc_vehicle_status mpc_vehicle_land_detected1 : BusAssignment  Commented=on  AssignedSignals=mpc_param_find
  select vxy : Selector  InputPortWidth=3  IndexOptions=Index vector (dialog)  Indices=[1 2]  OutputSizes=1
  select xy : Selector  InputPortWidth=3  IndexOptions=Index vector (dialog)  Indices=[1 2]  OutputSizes=1
  qDes : Outport  PortDimensions=4  SampleTime=MPC_SAMPLING_PERIOD
  thrustDes : Outport  Port=2  PortDimensions=1  SampleTime=MPC_SAMPLING_PERIOD
  yawRateDes : Outport  Port=3  PortDimensions=1  SampleTime=MPC_SAMPLING_PERIOD
  bus : Outport  Port=4  SampleTime=MPC_SAMPLING_PERIOD
  wires:
  mc_pos_control_main/1(selfOut) -> Unit Delay/1, bus/1, Bus Selector/1
  qNED/1 -> mpc_ctrl_state/3
  mpc_vehicle_status mpc_vehicle_land_detected/1 -> mpc_ctrl_state/1
  mpc_control_mode/1 -> mpc_manual/1
  mpc_ctrl_state/1 -> mpc_control_mode/1
  mpc_manual/1 -> mpc_arming/1
  mpc_arming/1 -> mpc_local_pos/1
  mpc_local_pos/1 -> mpc_pos_sp_triplet - current/1
  mpc_pos_sp_triplet - current/1 -> mpc_pos_sp_triplet - next/1
  mpc_pos_sp_triplet - next/1 -> mpc_pos_sp_triplet - previous/1
  mpc_pos_sp_triplet - previous/1 -> mpc_pos_sp_triplet - previous1/1
  Constant6/1 -> mpc_local_pos/24, mpc_local_pos/20, mpc_local_pos/18, mpc_local_pos/15
  Constant/1 -> mpc_local_pos/25, mpc_local_pos/8, mpc_local_pos/21
  Digital Clock/1 -> Gain/1
  Gain/1 -> [timestamp]
  [timestamp] -> mpc_local_pos/12, mpc_local_pos/13
  mpc_pos_sp_triplet - previous1/1 -> mc_pos_control_main/1(self)
  [timestamp] -> mpc_pos_sp_triplet - previous1/2
  Constant1/1 -> mpc_local_pos/9
  Constant3/1 -> mpc_local_pos/11
  Constant2/1 -> mpc_local_pos/10
  velNED/1 -> Demux/1, select vxy/1
  Demux/2 -> mpc_local_pos/16
  Demux/1 -> mpc_local_pos/14
  posNED/1 -> select xy/1, Demux1/1
  Demux1/1 -> mpc_local_pos/19
  Demux1/2 -> mpc_local_pos/22
  Gain4/1 -> mpc_local_pos/7
  Difference1/1 -> mpc_local_pos/5
  Difference/1 -> mpc_local_pos/3
  Difference2/1 -> mpc_local_pos/2
  select vxy/1 -> Difference2/1
  Difference3/1 -> mpc_local_pos/4
  select xy/1 -> Difference3/1
  Ground1/1 -> mpc_vehicle_status mpc_vehicle_land_detected/4, mpc_vehicle_status mpc_vehicle_land_detected/3, mpc_vehicle_status mpc_vehicle_land_detected/2
  Ground2/1 -> mpc_ctrl_state/4
  Constant4/1 -> mpc_control_mode/9, mpc_control_mode/10, mpc_control_mode/8, mpc_control_mode/6, mpc_control_mode/5, mpc_control_mode/4, mpc_control_mode/3
  Ground3/1 -> mpc_control_mode/7
  Ground4/1 -> mpc_manual/2
  stick/1 -> Demux2/1
  Demux2/1 -> mpc_manual/4
  Demux2/2 -> mpc_manual/5
  Demux2/3 -> mpc_manual/6
  Demux2/4 -> mpc_manual/3
  Ground5/1 -> mpc_pos_sp_triplet - current/3, mpc_pos_sp_triplet - current/5, mpc_pos_sp_triplet - current/6, mpc_pos_sp_triplet - current/7, mpc_pos_sp_triplet - current/8, mpc_pos_sp_triplet - current/9, mpc_pos_sp_triplet - current/10, mpc_pos_sp_triplet - current/11, mpc_pos_sp_triplet - current/12, mpc_pos_sp_triplet - current/13, mpc_pos_sp_triplet - current/14, mpc_pos_sp_triplet - current/15, mpc_pos_sp_triplet - current/16, mpc_pos_sp_triplet - current/17, mpc_pos_sp_triplet - current/18, mpc_pos_sp_triplet - current/19, mpc_pos_sp_triplet - current/20, mpc_pos_sp_triplet - current/21, mpc_pos_sp_triplet - current/22, mpc_pos_sp_triplet - current/23, mpc_pos_sp_triplet - current/24, mpc_pos_sp_triplet - current/25, mpc_pos_sp_triplet - current/26, mpc_pos_sp_triplet - current/27, mpc_pos_sp_triplet - current/4, mpc_pos_sp_triplet - current/2
  Ground6/1 -> mpc_pos_sp_triplet - next/5, mpc_pos_sp_triplet - next/4, mpc_pos_sp_triplet - next/3, mpc_pos_sp_triplet - next/2
  Ground7/1 -> mpc_pos_sp_triplet - previous/5, mpc_pos_sp_triplet - previous/4, mpc_pos_sp_triplet - previous/3, mpc_pos_sp_triplet - previous/2
  armed/1 -> [armed]
  [armed] -> mpc_arming/2
  [armed] -> mpc_control_mode/2
  Demux/3 -> mpc_local_pos/17, Difference/1, Gain4/1
  Constant5/1 -> mpc_ctrl_state/2
  Unit Delay/1 -> mpc_vehicle_status mpc_vehicle_land_detected/1
  Bus Creator/1 -> mpc_vehicle_status mpc_vehicle_land_detected1/2
  Demux3/1 -> Bus Creator/1
  Demux3/2 -> Bus Creator/2
  Demux3/3 -> Bus Creator/3
  Demux3/4 -> Bus Creator/4
  Demux3/5 -> Bus Creator/5
  Demux3/6 -> Bus Creator/6
  Demux3/7 -> Bus Creator/7
  Demux3/8 -> Bus Creator/8
  Demux3/9 -> Bus Creator/9
  Demux3/10 -> Bus Creator/10
  Demux3/11 -> Bus Creator/11
  Demux3/12 -> Bus Creator/12
  Demux3/13 -> Bus Creator/13
  Demux3/14 -> Bus Creator/14
  Demux3/15 -> Bus Creator/15
  Demux3/16 -> Bus Creator/16
  Demux3/17 -> Bus Creator/17
  Demux3/18 -> Bus Creator/18
  Demux3/19 -> Bus Creator/19
  Demux3/20 -> Bus Creator/20
  Demux3/21 -> Bus Creator/21
  Demux3/22 -> Bus Creator/22
  Demux3/23 -> Bus Creator/23
  Demux3/24 -> Bus Creator/24
  Demux3/25 -> Bus Creator/25
  Demux3/26 -> Bus Creator/26
  Demux3/27 -> Bus Creator/27
  Demux3/28 -> Bus Creator/28
  Demux3/29 -> Bus Creator/29
  Demux3/30 -> Bus Creator/30
  Demux3/31 -> Bus Creator/31
  Demux3/32 -> Bus Creator/32
  Demux3/33 -> Bus Creator/33
  Demux3/34 -> Bus Creator/34
  Constant7/1 -> Demux3/1
  Demux3/35 -> Bus Creator/35
  Demux1/3 -> mpc_local_pos/23, Gain1/1, Difference1/1
  Gain1/1 -> mpc_local_pos/6
  Bus Selector/3 -> yawRateDes/1  "<yaw_sp_move_rate>"
  Bus Selector/2 -> thrustDes/1  "<thrust>"
  Bus Selector/1 -> qDes/1  "<q_d>"

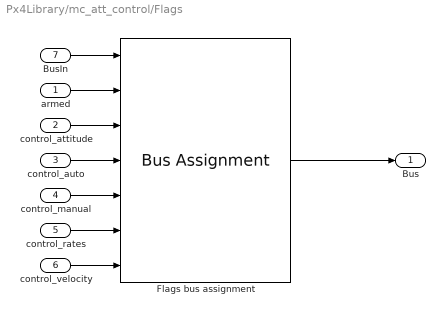
== system Px4Library/mc_att_control/Flags ==
  armed : Inport
  control_attitude : Inport  Port=2
  control_auto : Inport  Port=3
  control_manual : Inport  Port=4
  control_rates : Inport  Port=5
  control_velocity : Inport  Port=6
  BusIn : Inport  Port=7
  Flags bus assignment : BusAssignment  AssignedSignals=armed.armed,v_control_mode.flag_control_attitude_enabled,v_control_mode.flag_control_auto_enabled,v_control_mode.flag_control_manual_enabled,v_control_mode.flag_control_rates_enabled,v_control_mode.flag_control_velocity_enabled
  Bus : Outport
  wires:
  Flags bus assignment/1 -> Bus/1
  BusIn/1 -> Flags bus assignment/1
  control_auto/1 -> Flags bus assignment/4
  control_velocity/1 -> Flags bus assignment/7
  armed/1 -> Flags bus assignment/2
  control_attitude/1 -> Flags bus assignment/3
  control_manual/1 -> Flags bus assignment/5
  control_rates/1 -> Flags bus assignment/6

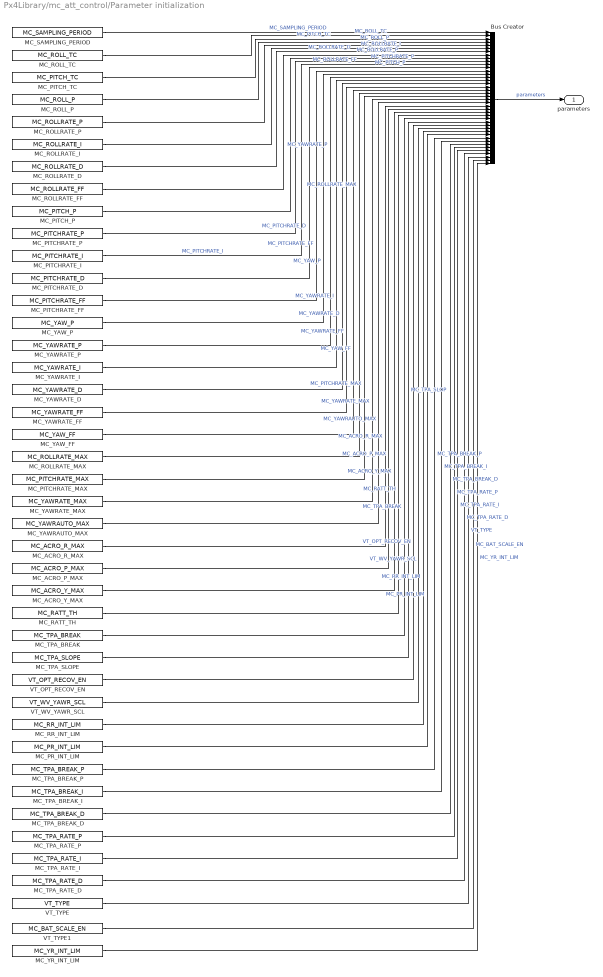
== system Px4Library/mc_att_control/Parameter initialization ==
  Bus Creator : BusCreator  Inputs='MC_SAMPLING_PERIOD','MC_ROLL_TC','MC_PITCH_TC','MC_ROLL_P','MC_ROLLRATE_P','MC_ROLLRATE_I','MC_ROLLRATE_D','MC_ROLLRATE_FF','MC_PITCH_P','MC_PITCHRATE_P','MC_PITCHRATE_I','MC_PITCHRATE_D','MC_PITCHRATE_FF','MC_YAW_P','MC_YAWRATE_P','MC_YAWRATE_I','MC_YAWRATE_D','MC_YAWRATE_FF','MC_YAW_FF','MC_ROLLRATE_MAX','MC_PITCHRATE_MAX','MC_YAWRATE_MAX','MC_YAWRAUTO_MAX','MC_ACRO_R_MAX','MC_ACRO_P_MAX','MC_ACRO_Y_MAX','MC_RATT_TH','MC_TPA_BREAK','MC_TPA_SLOP','VT_OPT_RECOV_EN','VT_WV_YAWR_SCL','MC_RR_INT_LIM','MC_PR_INT_LIM','MC_TPA_BREAK_P','MC_TPA_BREAK_I','MC_TPA_BREAK_D','MC_TPA_RATE_P','MC_TPA_RATE_I','MC_TPA_RATE_D','VT_TYPE','MC_BAT_SCALE_EN','MC_YR_INT_LIM'  OutDataTypeStr=Bus: parameterBus
  MC_ACRO_P_MAX : Constant  Value=MC_ACRO_P_MAX
  MC_ACRO_R_MAX : Constant  Value=MC_ACRO_R_MAX
  MC_ACRO_Y_MAX : Constant  Value=MC_ACRO_Y_MAX
  MC_PITCHRATE_D : Constant  Value=MC_PITCHRATE_D
  MC_PITCHRATE_FF : Constant  Value=MC_PITCHRATE_FF
  MC_PITCHRATE_I : Constant  Value=MC_PITCHRATE_I
  MC_PITCHRATE_MAX : Constant  Value=MC_PITCHRATE_MAX
  MC_PITCHRATE_P : Constant  Value=MC_PITCHRATE_P
  MC_PITCH_P : Constant  Value=MC_PITCH_P
  MC_PITCH_TC : Constant  Value=MC_PITCH_TC
  MC_PR_INT_LIM : Constant  Value=MC_PR_INT_LIM
  MC_RATT_TH : Constant  Value=MC_RATT_TH
  MC_ROLLRATE_D : Constant  Value=MC_ROLLRATE_D
  MC_ROLLRATE_FF : Constant  Value=MC_ROLLRATE_FF
  MC_ROLLRATE_I : Constant  Value=MC_ROLLRATE_I
  MC_ROLLRATE_MAX : Constant  Value=MC_ROLLRATE_MAX
  MC_ROLLRATE_P : Constant  Value=MC_ROLLRATE_P
  MC_ROLL_P : Constant  Value=MC_ROLL_P
  MC_ROLL_TC : Constant  Value=MC_ROLL_TC
  MC_RR_INT_LIM : Constant  Value=MC_RR_INT_LIM
  MC_SAMPLING_PERIOD : Constant  Value=MC_SAMPLING_PERIOD
  MC_TPA_BREAK : Constant  Value=MC_TPA_BREAK
  MC_TPA_BREAK_D : Constant  Value=MC_TPA_BREAK_D
  MC_TPA_BREAK_I : Constant  Value=MC_TPA_BREAK_I
  MC_TPA_BREAK_P : Constant  Value=MC_TPA_BREAK_P
  MC_TPA_RATE_D : Constant  Value=MC_TPA_RATE_D
  MC_TPA_RATE_I : Constant  Value=MC_TPA_RATE_I
  MC_TPA_RATE_P : Constant  Value=MC_TPA_RATE_P
  MC_TPA_SLOPE : Constant  Value=MC_TPA_SLOPE
  MC_YAWRATE_D : Constant  Value=MC_YAWRATE_D
  MC_YAWRATE_FF : Constant  Value=MC_YAWRATE_FF
  MC_YAWRATE_I : Constant  Value=MC_YAWRATE_I
  MC_YAWRATE_MAX : Constant  Value=MC_YAWRATE_MAX
  MC_YAWRATE_P : Constant  Value=MC_YAWRATE_P
  MC_YAWRAUTO_MAX : Constant  Value=MC_YAWRAUTO_MAX
  MC_YAW_FF : Constant  Value=MC_YAW_FF
  MC_YAW_P : Constant  Value=MC_YAW_P
  MC_YR_INT_LIM : Constant  Value=MC_YR_INT_LIM
  VT_OPT_RECOV_EN : Constant  Value=VT_OPT_RECOV_EN
  VT_TYPE : Constant  Value=VT_TYPE
  VT_TYPE1 : Constant  Value=MC_BAT_SCALE_EN
  VT_WV_YAWR_SCL : Constant  Value=VT_WV_YAWR_SCL
  parameters : Outport
  wires:
  MC_TPA_RATE_I/1 -> Bus Creator/38  "MC_TPA_RATE_I"
  MC_TPA_RATE_P/1 -> Bus Creator/37  "MC_TPA_RATE_P"
  MC_PR_INT_LIM/1 -> Bus Creator/33  "MC_PR_INT_LIM"
  MC_ROLLRATE_I/1 -> Bus Creator/6  "MC_ROLLRATE_I"
  MC_YAWRATE_D/1 -> Bus Creator/17  "MC_YAWRATE_D"
  MC_YAW_FF/1 -> Bus Creator/19  "MC_YAW_FF"
  MC_PITCHRATE_FF/1 -> Bus Creator/13  "MC_PITCHRATE_FF"
  MC_PITCHRATE_P/1 -> Bus Creator/10  "MC_PITCHRATE_P"
  MC_ROLLRATE_P/1 -> Bus Creator/5  "MC_ROLLRATE_P"
  MC_ROLLRATE_D/1 -> Bus Creator/7  "MC_ROLLRATE_D"
  MC_PITCHRATE_I/1 -> Bus Creator/11  "MC_PITCHRATE_I"
  MC_PITCHRATE_D/1 -> Bus Creator/12  "MC_PITCHRATE_D"
  MC_ROLLRATE_FF/1 -> Bus Creator/8  "MC_ROLLRATE_FF"
  MC_YAWRATE_FF/1 -> Bus Creator/18  "MC_YAWRATE_FF"
  MC_YAW_P/1 -> Bus Creator/14  "MC_YAW_P"
  MC_ROLLRATE_MAX/1 -> Bus Creator/20  "MC_ROLLRATE_MAX"
  MC_ROLL_P/1 -> Bus Creator/4  "MC_ROLL_P"
  MC_YAWRATE_I/1 -> Bus Creator/16  "MC_YAWRATE_I"
  MC_PITCHRATE_MAX/1 -> Bus Creator/21  "MC_PITCHRATE_MAX"
  MC_SAMPLING_PERIOD/1 -> Bus Creator/1  "MC_SAMPLING_PERIOD"
  MC_PITCH_TC/1 -> Bus Creator/3  "MC_PITCH_TC"
  MC_PITCH_P/1 -> Bus Creator/9  "MC_PITCH_P"
  MC_ROLL_TC/1 -> Bus Creator/2  "MC_ROLL_TC"
  MC_YAWRATE_P/1 -> Bus Creator/15  "MC_YAWRATE_P"
  MC_YAWRAUTO_MAX/1 -> Bus Creator/23  "MC_YAWRAUTO_MAX"
  MC_YAWRATE_MAX/1 -> Bus Creator/22  "MC_YAWRATE_MAX"
  MC_RATT_TH/1 -> Bus Creator/27  "MC_RATT_TH"
  VT_OPT_RECOV_EN/1 -> Bus Creator/30  "VT_OPT_RECOV_EN"
  MC_ACRO_Y_MAX/1 -> Bus Creator/26  "MC_ACRO_Y_MAX"
  MC_ACRO_P_MAX/1 -> Bus Creator/25  "MC_ACRO_P_MAX"
  Bus Creator/1 -> parameters/1  "parameters"
  MC_ACRO_R_MAX/1 -> Bus Creator/24  "MC_ACRO_R_MAX"
  MC_TPA_SLOPE/1 -> Bus Creator/29  "MC_TPA_SLOP"
  VT_WV_YAWR_SCL/1 -> Bus Creator/31  "VT_WV_YAWR_SCL"
  MC_TPA_BREAK/1 -> Bus Creator/28  "MC_TPA_BREAK"
  VT_TYPE/1 -> Bus Creator/40  "VT_TYPE"
  MC_TPA_RATE_D/1 -> Bus Creator/39  "MC_TPA_RATE_D"
  MC_YR_INT_LIM/1 -> Bus Creator/42  "MC_YR_INT_LIM"
  MC_TPA_BREAK_P/1 -> Bus Creator/34  "MC_TPA_BREAK_P"
  MC_TPA_BREAK_I/1 -> Bus Creator/35  "MC_TPA_BREAK_I"
  MC_TPA_BREAK_D/1 -> Bus Creator/36  "MC_TPA_BREAK_D"
  VT_TYPE1/1 -> Bus Creator/41  "MC_BAT_SCALE_EN"
  MC_RR_INT_LIM/1 -> Bus Creator/32  "MC_RR_INT_LIM"

== matlab function Px4Library/local_position_estimator/Input assignment ==
  data: armed_armed input; att_q input; mocap_timestamp input; mocap_updated input; mocap_x input; mocap_y input; mocap_z input; sensor_accelerometer_m_s2 input; sensor_baro_alt_meter input; sensor_baro_timestamp_relative input; sensor_timestamp input; sensor_updated input; selfVecIn input; selfVec output
function selfVec = InputAssignment( ...
	                             armed_armed, ...
	                                   att_q, ...
	                         mocap_timestamp, ...
	                           mocap_updated, ...
	                                 mocap_x, ...
	                                 mocap_y, ...
	                                 mocap_z, ...
	               sensor_accelerometer_m_s2, ...
	                   sensor_baro_alt_meter, ...
	          sensor_baro_timestamp_relative, ...
	                        sensor_timestamp, ...
	                          sensor_updated, ...
	                               selfVecIn ...
	)
%#codegen

	selfVec = selfVecIn;

	% Variable assignment
	selfVec(518:518) =                              armed_armed;
	selfVec(519:522) =                                    att_q;
	selfVec(530:530) =                          mocap_timestamp;
	selfVec(531:531) =                            mocap_updated;
	selfVec(532:532) =                                  mocap_x;
	selfVec(533:533) =                                  mocap_y;
	selfVec(534:534) =                                  mocap_z;
	selfVec(537:539) =                sensor_accelerometer_m_s2;
	selfVec(540:540) =                    sensor_baro_alt_meter;
	selfVec(541:541) =           sensor_baro_timestamp_relative;
	selfVec(542:542) =                         sensor_timestamp;
	selfVec(543:543) =                           sensor_updated;
end
